simulink library "lib_BuildingThermalLiquid"  (R2026a)
settings: Solver=VariableStepAuto
libraries: ExternalWall_lib x47, WallSelector_lib x36, fl_lib x20, RoomWithRadiatorAndUFP x15
(part 1 of 5)
settings Model: Creator=vikrants  LastModifiedBy=vikrants

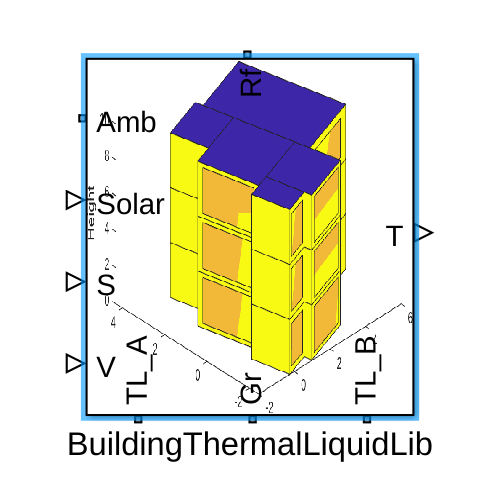
[thumbnail: Simulink's stored preview of the top-level diagram]
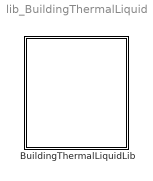
== system lib_BuildingThermalLiquid ==
  BuildingThermalLiquidLib : Subsystem
      settings: PortSchema="{\"entries\":[{\"content\":{\"sides\":[{\"content\":{\"connectorIds\":[\"LConn1\",\"LConn2\",\"LConn3\",\"LConn4\"]},\"type\":\"ConnectorPlacement.EquallySpacedRectSide\",\"uuid\":\"3d4f604e-be28-4e36-924c-1451eaa25fd5\"},{\"content\":{\"connectorIds\":[\"RConn1\"],\"side\":\"RIGHT\"},\"type\":\"ConnectorPlacement.EquallySpacedRectSide\",\"uuid\":\"4c994dcc-0f2c-417a-aef1-7383a3b9052f\"},{\"content\":{\"connectorIds\":[\"LConn5\"],\"side\":\"TOP\"},\"type\":\"ConnectorPlacement.EquallySpacedRectSide\",\"uuid\":\"8e95fada-93f8-47aa-9321-3e2d1640391a\"},{\"content\":{\"connectorIds\":[\"RConn2\",\"RConn3\",\"RConn4\"],\"side\":\"BOTTOM\"},\"type\":\"ConnectorPlacement.EquallySpacedRectSide\",\"uuid\":\"74174f52-ffa4-469a-aac5-7e57a56dc597\"}]},\"type\":\"ConnectorPlacement.EquallySpacedConnector\",\"uuid\":\"f223b6b9-b787-430f-8486-49686756d9cb\"}],\"packageUris\":[\"http://schema.mathworks.com/mf0/Connector/R2020b\"],\"version\":\"1.0\"}"
      mask Display: image('lib_BuildingThermalLiquid.png')

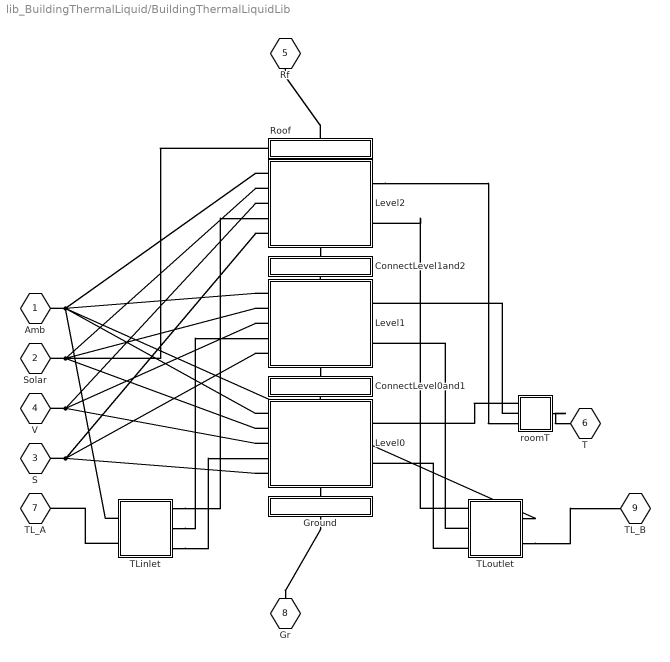
== system lib_BuildingThermalLiquid/BuildingThermalLiquidLib ==
  ConnectLevel0and1 : Subsystem
      settings: PortSchema="{\"entries\":[{\"content\":{\"sides\":[{\"content\":{},\"type\":\"ConnectorPlacement.EquallySpacedRectSide\",\"uuid\":\"f2497a14-4137-415a-aa8b-f8737c2b6cdd\"},{\"content\":{\"side\":\"RIGHT\"},\"type\":\"ConnectorPlacement.EquallySpacedRectSide\",\"uuid\":\"642fe1c4-bc52-48dc-8376-fc1f54abf874\"},{\"content\":{\"connectorIds\":[\"LConn1\"],\"side\":\"TOP\"},\"type\":\"ConnectorPlacement.EquallySpacedRectSide\",\"uuid\":\"0041873e-f83c-4980-a922-5fb2e99c62be\"},{\"content\":{\"connectorIds\":[\"RConn1\"],\"side\":\"BOTTOM\"},\"type\":\"ConnectorPlacement.EquallySpacedRectSide\",\"uuid\":\"519cd5c6-7a50-4e8d-a798-15261cf86acb\"}]},\"type\":\"ConnectorPlacement.EquallySpacedConnector\",\"uuid\":\"f9a0d06d-e057-47b8-97bb-81916403e866\"}],\"packageUris\":[\"http://schema.mathworks.com/mf0/Connector/R2020b\"],\"version\":\"1.0\"}"
  ConnectLevel1and2 : Subsystem
      settings: PortSchema="{\"entries\":[{\"content\":{\"sides\":[{\"content\":{},\"type\":\"ConnectorPlacement.EquallySpacedRectSide\",\"uuid\":\"f2497a14-4137-415a-aa8b-f8737c2b6cdd\"},{\"content\":{\"side\":\"RIGHT\"},\"type\":\"ConnectorPlacement.EquallySpacedRectSide\",\"uuid\":\"642fe1c4-bc52-48dc-8376-fc1f54abf874\"},{\"content\":{\"connectorIds\":[\"LConn1\"],\"side\":\"TOP\"},\"type\":\"ConnectorPlacement.EquallySpacedRectSide\",\"uuid\":\"0041873e-f83c-4980-a922-5fb2e99c62be\"},{\"content\":{\"connectorIds\":[\"RConn1\"],\"side\":\"BOTTOM\"},\"type\":\"ConnectorPlacement.EquallySpacedRectSide\",\"uuid\":\"a780114b-2d0a-4cf5-8292-ebaab293840d\"}]},\"type\":\"ConnectorPlacement.EquallySpacedConnector\",\"uuid\":\"f9a0d06d-e057-47b8-97bb-81916403e866\"}],\"packageUris\":[\"http://schema.mathworks.com/mf0/Connector/R2020b\"],\"version\":\"1.0\"}"
  Ground : Subsystem
      settings: PortSchema="{\"entries\":[{\"content\":{\"sides\":[{\"content\":{},\"type\":\"ConnectorPlacement.EquallySpacedRectSide\",\"uuid\":\"f2497a14-4137-415a-aa8b-f8737c2b6cdd\"},{\"content\":{\"side\":\"RIGHT\"},\"type\":\"ConnectorPlacement.EquallySpacedRectSide\",\"uuid\":\"642fe1c4-bc52-48dc-8376-fc1f54abf874\"},{\"content\":{\"connectorIds\":[\"LConn1\"],\"side\":\"TOP\"},\"type\":\"ConnectorPlacement.EquallySpacedRectSide\",\"uuid\":\"0041873e-f83c-4980-a922-5fb2e99c62be\"},{\"content\":{\"connectorIds\":[\"RConn1\"],\"side\":\"BOTTOM\"},\"type\":\"ConnectorPlacement.EquallySpacedRectSide\",\"uuid\":\"6efa04cd-1264-4f10-80b2-069a220ffbe0\"}]},\"type\":\"ConnectorPlacement.EquallySpacedConnector\",\"uuid\":\"f9a0d06d-e057-47b8-97bb-81916403e866\"}],\"packageUris\":[\"http://schema.mathworks.com/mf0/Connector/R2020b\"],\"version\":\"1.0\"}"
  Level0 : Subsystem
      settings: PortSchema="{\"entries\":[{\"content\":{\"sides\":[{\"content\":{\"connectorIds\":[\"LConn1\",\"LConn2\",\"LConn3\",\"LConn4\",\"LConn5\"]},\"type\":\"ConnectorPlacement.EquallySpacedRectSide\",\"uuid\":\"29492f5e-f304-4ed0-9062-38da432019c8\"},{\"content\":{\"connectorIds\":[\"RConn1\",\"RConn2\"],\"side\":\"RIGHT\"},\"type\":\"ConnectorPlacement.EquallySpacedRectSide\",\"uuid\":\"f46545ef-22ad-458b-9be7-cff6591fe741\"},{\"content\":{\"connectorIds\":[\"LConn6\"],\"side\":\"TOP\"},\"type\":\"ConnectorPlacement.EquallySpacedRectSide\",\"uuid\":\"9b1b30be-62a1-4a86-b987-44a9b36d130d\"},{\"content\":{\"connectorIds\":[\"RConn3\"],\"side\":\"BOTTOM\"},\"type\":\"ConnectorPlacement.EquallySpacedRectSide\",\"uuid\":\"1c461fab-c590-4319-ab41-1586157498f8\"}]},\"type\":\"ConnectorPlacement.EquallySpacedConnector\",\"uuid\":\"6c3f86bb-1201-4f27-98f2-2151c6075667\"}],\"packageUris\":[\"http://schema.mathworks.com/mf0/Connector/R2020b\"],\"version\":\"1.0\"}"
  Level1 : Subsystem
      settings: PortSchema="{\"entries\":[{\"content\":{\"sides\":[{\"content\":{\"connectorIds\":[\"LConn1\",\"LConn2\",\"LConn3\",\"LConn4\",\"LConn5\"]},\"type\":\"ConnectorPlacement.EquallySpacedRectSide\",\"uuid\":\"29492f5e-f304-4ed0-9062-38da432019c8\"},{\"content\":{\"connectorIds\":[\"RConn1\",\"RConn2\"],\"side\":\"RIGHT\"},\"type\":\"ConnectorPlacement.EquallySpacedRectSide\",\"uuid\":\"f46545ef-22ad-458b-9be7-cff6591fe741\"},{\"content\":{\"connectorIds\":[\"LConn6\"],\"side\":\"TOP\"},\"type\":\"ConnectorPlacement.EquallySpacedRectSide\",\"uuid\":\"9b1b30be-62a1-4a86-b987-44a9b36d130d\"},{\"content\":{\"connectorIds\":[\"RConn3\"],\"side\":\"BOTTOM\"},\"type\":\"ConnectorPlacement.EquallySpacedRectSide\",\"uuid\":\"e01c8120-d70d-4a42-a08e-230c171c29be\"}]},\"type\":\"ConnectorPlacement.EquallySpacedConnector\",\"uuid\":\"6c3f86bb-1201-4f27-98f2-2151c6075667\"}],\"packageUris\":[\"http://schema.mathworks.com/mf0/Connector/R2020b\"],\"version\":\"1.0\"}"
  Level2 : Subsystem
      settings: PortSchema="{\"entries\":[{\"content\":{\"sides\":[{\"content\":{\"connectorIds\":[\"LConn1\",\"LConn2\",\"LConn3\",\"LConn4\",\"LConn5\"]},\"type\":\"ConnectorPlacement.EquallySpacedRectSide\",\"uuid\":\"29492f5e-f304-4ed0-9062-38da432019c8\"},{\"content\":{\"connectorIds\":[\"RConn1\",\"RConn2\"],\"side\":\"RIGHT\"},\"type\":\"ConnectorPlacement.EquallySpacedRectSide\",\"uuid\":\"f46545ef-22ad-458b-9be7-cff6591fe741\"},{\"content\":{\"connectorIds\":[\"LConn6\"],\"side\":\"TOP\"},\"type\":\"ConnectorPlacement.EquallySpacedRectSide\",\"uuid\":\"9b1b30be-62a1-4a86-b987-44a9b36d130d\"},{\"content\":{\"connectorIds\":[\"RConn3\"],\"side\":\"BOTTOM\"},\"type\":\"ConnectorPlacement.EquallySpacedRectSide\",\"uuid\":\"fba86260-54d8-4078-9f73-b7a4e9f151fe\"}]},\"type\":\"ConnectorPlacement.EquallySpacedConnector\",\"uuid\":\"6c3f86bb-1201-4f27-98f2-2151c6075667\"}],\"packageUris\":[\"http://schema.mathworks.com/mf0/Connector/R2020b\"],\"version\":\"1.0\"}"
  Roof : Subsystem
      settings: PortSchema="{\"entries\":[{\"content\":{\"sides\":[{\"content\":{\"connectorIds\":[\"LConn1\"]},\"type\":\"ConnectorPlacement.EquallySpacedRectSide\",\"uuid\":\"8a3f7f62-740f-4024-84fd-cea985b0aa8d\"},{\"content\":{\"side\":\"RIGHT\"},\"type\":\"ConnectorPlacement.EquallySpacedRectSide\",\"uuid\":\"b896e2bb-4320-404c-bfaa-2c8ea40bf71f\"},{\"content\":{\"connectorIds\":[\"LConn2\"],\"side\":\"TOP\"},\"type\":\"ConnectorPlacement.EquallySpacedRectSide\",\"uuid\":\"76c3d6f3-9638-4345-911f-6db02cf3c8d9\"},{\"content\":{\"connectorIds\":[\"RConn1\"],\"side\":\"BOTTOM\"},\"type\":\"ConnectorPlacement.EquallySpacedRectSide\",\"uuid\":\"d013c520-b3cf-4758-8021-0d51b5bea7ff\"}]},\"type\":\"ConnectorPlacement.EquallySpacedConnector\",\"uuid\":\"2675eef2-482a-4a5a-91dc-eba58fd9f740\"}],\"packageUris\":[\"http://schema.mathworks.com/mf0/Connector/R2020b\"],\"version\":\"1.0\"}"
  TLinlet : Subsystem
  TLoutlet : Subsystem
  roomT : Subsystem
  Amb : PMIOPort  Side=Left
  Solar : PMIOPort  Port=2  Side=Left
  S : PMIOPort  Port=3  Side=Left
  V : PMIOPort  Port=4  Side=Left
  Rf : PMIOPort  Port=5  Side=Left
  T : PMIOPort  Port=6  Side=Right
  TL_A : PMIOPort  Port=7  Side=Right
  Gr : PMIOPort  Port=8  Side=Right
  TL_B : PMIOPort  Port=9  Side=Right
  connections:
  TLinlet/RConn1 -- Level2/LConn4
  TLoutlet/LConn1 -- Level2/RConn2
  TLinlet/RConn2 -- Level1/LConn4
  TLoutlet/LConn2 -- Level1/RConn2
  TLinlet/RConn3 -- Level0/LConn4
  TLoutlet/LConn3 -- Level0/RConn2
  Level0/RConn3 -- Ground/LConn1
  Level1/RConn3 -- ConnectLevel0and1/LConn1
  Level0/LConn6 -- ConnectLevel0and1/RConn1
  Level2/RConn3 -- ConnectLevel1and2/LConn1
  Level1/LConn6 -- ConnectLevel1and2/RConn1
  Level2/LConn6 -- Roof/RConn1
  Roof/LConn2 -- Rf/RConn1
  Ground/RConn1 -- Gr/RConn1
  Roof/LConn1 -- Solar/RConn1 -- Level2/LConn2 -- Level1/LConn2 -- Level0/LConn2
  Level0/LConn1 -- Amb/RConn1 -- TLoutlet/RConn1 -- TLinlet/LConn1 -- Level2/LConn1 -- Level1/LConn1
  Level0/LConn3 -- V/RConn1 -- Level2/LConn3 -- Level1/LConn3
  Level0/LConn5 -- S/RConn1 -- Level2/LConn5 -- Level1/LConn5
  TLinlet/LConn2 -- TL_A/RConn1
  TLoutlet/RConn2 -- TL_B/RConn1
  roomT/LConn2 -- Level1/RConn1
  roomT/RConn1 -- T/RConn1
  roomT/LConn1 -- Level0/RConn1
  Level2/RConn1 -- roomT/LConn3

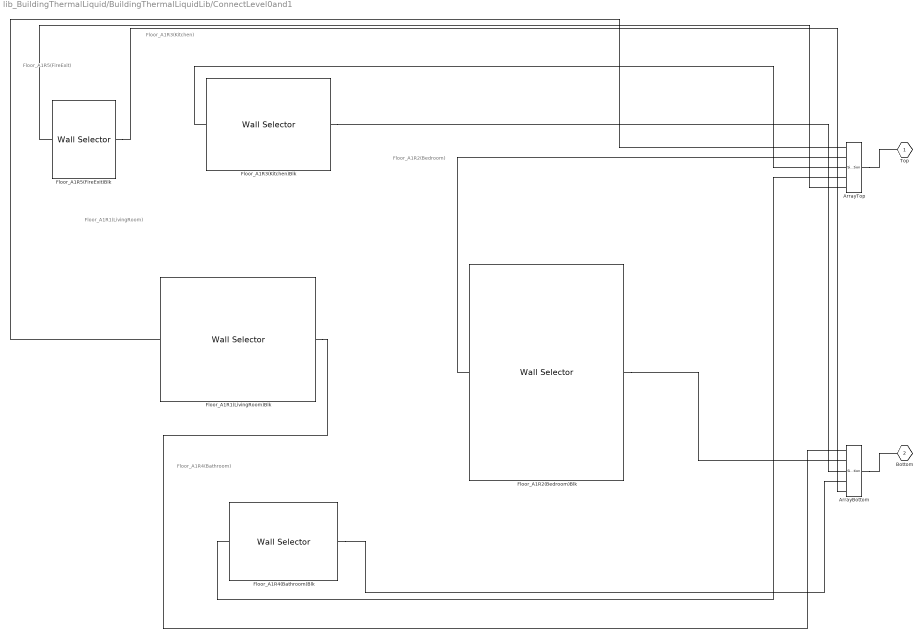
== system lib_BuildingThermalLiquid/BuildingThermalLiquidLib/ConnectLevel0and1 ==
  note: Floor_A1R1(LivingRoom)
  note: Floor_A1R2(Bedroom)
  note: Floor_A1R3(Kitchen)
  note: Floor_A1R4(Bathroom)
  note: Floor_A1R5(FireExit)
  ArrayBottom : SimscapeArrayConnection  Domain=foundation.thermal.thermal  ConcatenateDimension=1  NumScalarElements=5
  ArrayTop : SimscapeArrayConnection  Domain=foundation.thermal.thermal  ConcatenateDimension=1  NumScalarElements=5
  Floor_A1R1(LivingRoom)Blk : WallSelector_lib/Wall Selector  optWall=wallModelOption.wallOnly  wallLength=2.4384 % Parameterized on : 11-Dec-2025 09:25:46 m  wallHeight=3.048 % Parameterized on : 11-Dec-2025 09:25:46 m  wallThickness=0.03 % Parameterized on : 11-Dec-2025 09:25:46 m  wallMaterialDen=1400 % Parameterized on : 11-Dec-2025 09:25:49 kg/m^3  wallMaterialCp=1000 % Parameterized on : 11-Dec-2025 09:25:49 J/(K*kg)  wallAbsorptivity=0.5  wallThermalK=0.7 % Parameterized on : 11-Dec-2025 09:25:49 W/(K*m)  winLength=1 m  winHeight=0.5 m  winThickness=0.007 m  winMaterialDen=2500 kg/m^3  winMaterialCp=787 J/(K*kg)  winAbsorptivity=0.35  winThermalK=1 W/(K*m)  winTransmissivity=0.45  ventLength=0.1 m  ventHeight=0.1 m  extToWallHTC=30 % Parameterized on : 11-Dec-2025 09:25:49 W/(K*m^2)  intToRoomHTC=30 % Parameterized on : 11-Dec-2025 09:25:49 W/(K*m^2)  iniT=300 % Parameterized on : 11-Dec-2025 09:25:49 K
  Floor_A1R2(Bedroom)Blk : WallSelector_lib/Wall Selector  optWall=wallModelOption.wallOnly  wallLength=4.2672 % Parameterized on : 11-Dec-2025 09:25:46 m  wallHeight=3.048 % Parameterized on : 11-Dec-2025 09:25:46 m  wallThickness=0.03 % Parameterized on : 11-Dec-2025 09:25:46 m  wallMaterialDen=1400 % Parameterized on : 11-Dec-2025 09:25:49 kg/m^3  wallMaterialCp=1000 % Parameterized on : 11-Dec-2025 09:25:49 J/(K*kg)  wallAbsorptivity=0.5  wallThermalK=0.7 % Parameterized on : 11-Dec-2025 09:25:49 W/(K*m)  winLength=1 m  winHeight=0.5 m  winThickness=0.007 m  winMaterialDen=2500 kg/m^3  winMaterialCp=787 J/(K*kg)  winAbsorptivity=0.35  winThermalK=1 W/(K*m)  winTransmissivity=0.45  ventLength=0.1 m  ventHeight=0.1 m  extToWallHTC=30 % Parameterized on : 11-Dec-2025 09:25:49 W/(K*m^2)  intToRoomHTC=30 % Parameterized on : 11-Dec-2025 09:25:49 W/(K*m^2)  iniT=300 % Parameterized on : 11-Dec-2025 09:25:49 K
  Floor_A1R3(Kitchen)Blk : WallSelector_lib/Wall Selector  optWall=wallModelOption.wallOnly  wallLength=1.8288 % Parameterized on : 11-Dec-2025 09:25:46 m  wallHeight=2.4384 % Parameterized on : 11-Dec-2025 09:25:46 m  wallThickness=0.03 % Parameterized on : 11-Dec-2025 09:25:46 m  wallMaterialDen=1400 % Parameterized on : 11-Dec-2025 09:25:49 kg/m^3  wallMaterialCp=1000 % Parameterized on : 11-Dec-2025 09:25:49 J/(K*kg)  wallAbsorptivity=0.5  wallThermalK=0.7 % Parameterized on : 11-Dec-2025 09:25:49 W/(K*m)  winLength=1 m  winHeight=0.5 m  winThickness=0.007 m  winMaterialDen=2500 kg/m^3  winMaterialCp=787 J/(K*kg)  winAbsorptivity=0.35  winThermalK=1 W/(K*m)  winTransmissivity=0.45  ventLength=0.1 m  ventHeight=0.1 m  extToWallHTC=30 % Parameterized on : 11-Dec-2025 09:25:49 W/(K*m^2)  intToRoomHTC=30 % Parameterized on : 11-Dec-2025 09:25:49 W/(K*m^2)  iniT=300 % Parameterized on : 11-Dec-2025 09:25:49 K
  Floor_A1R4(Bathroom)Blk : WallSelector_lib/Wall Selector  optWall=wallModelOption.wallOnly  wallLength=1.524 % Parameterized on : 11-Dec-2025 09:25:46 m  wallHeight=2.1336 % Parameterized on : 11-Dec-2025 09:25:47 m  wallThickness=0.03 % Parameterized on : 11-Dec-2025 09:25:47 m  wallMaterialDen=1400 % Parameterized on : 11-Dec-2025 09:25:49 kg/m^3  wallMaterialCp=1000 % Parameterized on : 11-Dec-2025 09:25:49 J/(K*kg)  wallAbsorptivity=0.5  wallThermalK=0.7 % Parameterized on : 11-Dec-2025 09:25:49 W/(K*m)  winLength=1 m  winHeight=0.5 m  winThickness=0.007 m  winMaterialDen=2500 kg/m^3  winMaterialCp=787 J/(K*kg)  winAbsorptivity=0.35  winThermalK=1 W/(K*m)  winTransmissivity=0.45  ventLength=0.1 m  ventHeight=0.1 m  extToWallHTC=30 % Parameterized on : 11-Dec-2025 09:25:49 W/(K*m^2)  intToRoomHTC=30 % Parameterized on : 11-Dec-2025 09:25:49 W/(K*m^2)  iniT=300 % Parameterized on : 11-Dec-2025 09:25:49 K
  Floor_A1R5(FireExit)Blk : WallSelector_lib/Wall Selector  optWall=wallModelOption.wallOnly  wallLength=1.524 % Parameterized on : 11-Dec-2025 09:25:47 m  wallHeight=1.2192 % Parameterized on : 11-Dec-2025 09:25:47 m  wallThickness=0.03 % Parameterized on : 11-Dec-2025 09:25:47 m  wallMaterialDen=1400 % Parameterized on : 11-Dec-2025 09:25:49 kg/m^3  wallMaterialCp=1000 % Parameterized on : 11-Dec-2025 09:25:49 J/(K*kg)  wallAbsorptivity=0.5  wallThermalK=0.7 % Parameterized on : 11-Dec-2025 09:25:49 W/(K*m)  winLength=1 m  winHeight=0.5 m  winThickness=0.007 m  winMaterialDen=2500 kg/m^3  winMaterialCp=787 J/(K*kg)  winAbsorptivity=0.35  winThermalK=1 W/(K*m)  winTransmissivity=0.45  ventLength=0.1 m  ventHeight=0.1 m  extToWallHTC=30 % Parameterized on : 11-Dec-2025 09:25:49 W/(K*m^2)  intToRoomHTC=30 % Parameterized on : 11-Dec-2025 09:25:49 W/(K*m^2)  iniT=300 % Parameterized on : 11-Dec-2025 09:25:49 K
  Top : PMIOPort  Side=Left
  Bottom : PMIOPort  Port=2  Side=Right
  connections:
  ArrayTop/RConn1 -- Top/RConn1
  Floor_A1R1(LivingRoom)Blk/LConn1 -- ArrayTop/LConn1
  Floor_A1R2(Bedroom)Blk/LConn1 -- ArrayTop/LConn2
  Floor_A1R3(Kitchen)Blk/LConn1 -- ArrayTop/LConn3
  Floor_A1R4(Bathroom)Blk/LConn1 -- ArrayTop/LConn4
  Floor_A1R5(FireExit)Blk/LConn1 -- ArrayTop/LConn5
  ArrayBottom/RConn1 -- Bottom/RConn1
  Floor_A1R1(LivingRoom)Blk/RConn1 -- ArrayBottom/LConn1
  Floor_A1R2(Bedroom)Blk/RConn1 -- ArrayBottom/LConn2
  Floor_A1R3(Kitchen)Blk/RConn1 -- ArrayBottom/LConn3
  Floor_A1R4(Bathroom)Blk/RConn1 -- ArrayBottom/LConn4
  Floor_A1R5(FireExit)Blk/RConn1 -- ArrayBottom/LConn5

== system lib_BuildingThermalLiquid/BuildingThermalLiquidLib/ConnectLevel1and2 ==
  note: Floor_A2R1(LivingRoom)
  note: Floor_A2R2(Bedroom)
  note: Floor_A2R3(Kitchen)
  note: Floor_A2R4(Bathroom)
  note: Floor_A2R5(FireExit)
  ArrayBottom : SimscapeArrayConnection  Domain=foundation.thermal.thermal  ConcatenateDimension=1  NumScalarElements=5
  ArrayTop : SimscapeArrayConnection  Domain=foundation.thermal.thermal  ConcatenateDimension=1  NumScalarElements=5
  Floor_A2R1(LivingRoom)Blk : WallSelector_lib/Wall Selector  optWall=wallModelOption.wallOnly  wallLength=2.4384 % Parameterized on : 11-Dec-2025 09:25:47 m  wallHeight=3.048 % Parameterized on : 11-Dec-2025 09:25:47 m  wallThickness=0.03 % Parameterized on : 11-Dec-2025 09:25:47 m  wallMaterialDen=1400 % Parameterized on : 11-Dec-2025 09:25:49 kg/m^3  wallMaterialCp=1000 % Parameterized on : 11-Dec-2025 09:25:49 J/(K*kg)  wallAbsorptivity=0.5  wallThermalK=0.7 % Parameterized on : 11-Dec-2025 09:25:49 W/(K*m)  winLength=1 m  winHeight=0.5 m  winThickness=0.007 m  winMaterialDen=2500 kg/m^3  winMaterialCp=787 J/(K*kg)  winAbsorptivity=0.35  winThermalK=1 W/(K*m)  winTransmissivity=0.45  ventLength=0.1 m  ventHeight=0.1 m  extToWallHTC=30 % Parameterized on : 11-Dec-2025 09:25:49 W/(K*m^2)  intToRoomHTC=30 % Parameterized on : 11-Dec-2025 09:25:49 W/(K*m^2)  iniT=300 % Parameterized on : 11-Dec-2025 09:25:49 K
  Floor_A2R2(Bedroom)Blk : WallSelector_lib/Wall Selector  optWall=wallModelOption.wallOnly  wallLength=4.2672 % Parameterized on : 11-Dec-2025 09:25:47 m  wallHeight=3.048 % Parameterized on : 11-Dec-2025 09:25:47 m  wallThickness=0.03 % Parameterized on : 11-Dec-2025 09:25:47 m  wallMaterialDen=1400 % Parameterized on : 11-Dec-2025 09:25:49 kg/m^3  wallMaterialCp=1000 % Parameterized on : 11-Dec-2025 09:25:49 J/(K*kg)  wallAbsorptivity=0.5  wallThermalK=0.7 % Parameterized on : 11-Dec-2025 09:25:49 W/(K*m)  winLength=1 m  winHeight=0.5 m  winThickness=0.007 m  winMaterialDen=2500 kg/m^3  winMaterialCp=787 J/(K*kg)  winAbsorptivity=0.35  winThermalK=1 W/(K*m)  winTransmissivity=0.45  ventLength=0.1 m  ventHeight=0.1 m  extToWallHTC=30 % Parameterized on : 11-Dec-2025 09:25:49 W/(K*m^2)  intToRoomHTC=30 % Parameterized on : 11-Dec-2025 09:25:49 W/(K*m^2)  iniT=300 % Parameterized on : 11-Dec-2025 09:25:49 K
  Floor_A2R3(Kitchen)Blk : WallSelector_lib/Wall Selector  optWall=wallModelOption.wallOnly  wallLength=1.8288 % Parameterized on : 11-Dec-2025 09:25:47 m  wallHeight=2.4384 % Parameterized on : 11-Dec-2025 09:25:47 m  wallThickness=0.03 % Parameterized on : 11-Dec-2025 09:25:47 m  wallMaterialDen=1400 % Parameterized on : 11-Dec-2025 09:25:49 kg/m^3  wallMaterialCp=1000 % Parameterized on : 11-Dec-2025 09:25:49 J/(K*kg)  wallAbsorptivity=0.5  wallThermalK=0.7 % Parameterized on : 11-Dec-2025 09:25:49 W/(K*m)  winLength=1 m  winHeight=0.5 m  winThickness=0.007 m  winMaterialDen=2500 kg/m^3  winMaterialCp=787 J/(K*kg)  winAbsorptivity=0.35  winThermalK=1 W/(K*m)  winTransmissivity=0.45  ventLength=0.1 m  ventHeight=0.1 m  extToWallHTC=30 % Parameterized on : 11-Dec-2025 09:25:49 W/(K*m^2)  intToRoomHTC=30 % Parameterized on : 11-Dec-2025 09:25:49 W/(K*m^2)  iniT=300 % Parameterized on : 11-Dec-2025 09:25:49 K
  Floor_A2R4(Bathroom)Blk : WallSelector_lib/Wall Selector  optWall=wallModelOption.wallOnly  wallLength=1.524 % Parameterized on : 11-Dec-2025 09:25:47 m  wallHeight=2.1336 % Parameterized on : 11-Dec-2025 09:25:47 m  wallThickness=0.03 % Parameterized on : 11-Dec-2025 09:25:47 m  wallMaterialDen=1400 % Parameterized on : 11-Dec-2025 09:25:49 kg/m^3  wallMaterialCp=1000 % Parameterized on : 11-Dec-2025 09:25:49 J/(K*kg)  wallAbsorptivity=0.5  wallThermalK=0.7 % Parameterized on : 11-Dec-2025 09:25:49 W/(K*m)  winLength=1 m  winHeight=0.5 m  winThickness=0.007 m  winMaterialDen=2500 kg/m^3  winMaterialCp=787 J/(K*kg)  winAbsorptivity=0.35  winThermalK=1 W/(K*m)  winTransmissivity=0.45  ventLength=0.1 m  ventHeight=0.1 m  extToWallHTC=30 % Parameterized on : 11-Dec-2025 09:25:49 W/(K*m^2)  intToRoomHTC=30 % Parameterized on : 11-Dec-2025 09:25:49 W/(K*m^2)  iniT=300 % Parameterized on : 11-Dec-2025 09:25:49 K
  Floor_A2R5(FireExit)Blk : WallSelector_lib/Wall Selector  optWall=wallModelOption.wallOnly  wallLength=1.524 % Parameterized on : 11-Dec-2025 09:25:47 m  wallHeight=1.2192 % Parameterized on : 11-Dec-2025 09:25:47 m  wallThickness=0.03 % Parameterized on : 11-Dec-2025 09:25:47 m  wallMaterialDen=1400 % Parameterized on : 11-Dec-2025 09:25:49 kg/m^3  wallMaterialCp=1000 % Parameterized on : 11-Dec-2025 09:25:49 J/(K*kg)  wallAbsorptivity=0.5  wallThermalK=0.7 % Parameterized on : 11-Dec-2025 09:25:49 W/(K*m)  winLength=1 m  winHeight=0.5 m  winThickness=0.007 m  winMaterialDen=2500 kg/m^3  winMaterialCp=787 J/(K*kg)  winAbsorptivity=0.35  winThermalK=1 W/(K*m)  winTransmissivity=0.45  ventLength=0.1 m  ventHeight=0.1 m  extToWallHTC=30 % Parameterized on : 11-Dec-2025 09:25:49 W/(K*m^2)  intToRoomHTC=30 % Parameterized on : 11-Dec-2025 09:25:49 W/(K*m^2)  iniT=300 % Parameterized on : 11-Dec-2025 09:25:49 K
  Top : PMIOPort  Side=Left
  Bottom : PMIOPort  Port=2  Side=Right
  connections:
  ArrayTop/RConn1 -- Top/RConn1
  Floor_A2R1(LivingRoom)Blk/LConn1 -- ArrayTop/LConn1
  Floor_A2R2(Bedroom)Blk/LConn1 -- ArrayTop/LConn2
  Floor_A2R3(Kitchen)Blk/LConn1 -- ArrayTop/LConn3
  Floor_A2R4(Bathroom)Blk/LConn1 -- ArrayTop/LConn4
  Floor_A2R5(FireExit)Blk/LConn1 -- ArrayTop/LConn5
  ArrayBottom/RConn1 -- Bottom/RConn1
  Floor_A2R1(LivingRoom)Blk/RConn1 -- ArrayBottom/LConn1
  Floor_A2R2(Bedroom)Blk/RConn1 -- ArrayBottom/LConn2
  Floor_A2R3(Kitchen)Blk/RConn1 -- ArrayBottom/LConn3
  Floor_A2R4(Bathroom)Blk/RConn1 -- ArrayBottom/LConn4
  Floor_A2R5(FireExit)Blk/RConn1 -- ArrayBottom/LConn5

== system lib_BuildingThermalLiquid/BuildingThermalLiquidLib/Ground ==
  note: Ground_A1R1(LivingRoom)
  note: Ground_A1R2(Bedroom)
  note: Ground_A1R3(Kitchen)
  note: Ground_A1R4(Bathroom)
  note: Ground_A1R5(FireExit)
  ArrayBottom : SimscapeArrayConnection  Domain=foundation.thermal.thermal  ConcatenateDimension=1  NumScalarElements=5
  ArrayTop : SimscapeArrayConnection  Domain=foundation.thermal.thermal  ConcatenateDimension=1  NumScalarElements=5
  Ground_A1R1(LivingRoom)Blk : WallSelector_lib/Wall Selector  optWall=wallModelOption.wallOnly  wallLength=2.4384 % Parameterized on : 11-Dec-2025 09:25:47 m  wallHeight=3.048 % Parameterized on : 11-Dec-2025 09:25:47 m  wallThickness=0.03 % Parameterized on : 11-Dec-2025 09:25:47 m  wallMaterialDen=1400 % Parameterized on : 11-Dec-2025 09:25:49 kg/m^3  wallMaterialCp=1000 % Parameterized on : 11-Dec-2025 09:25:49 J/(K*kg)  wallAbsorptivity=0.5  wallThermalK=0.7 % Parameterized on : 11-Dec-2025 09:25:49 W/(K*m)  winLength=1 m  winHeight=0.5 m  winThickness=0.007 m  winMaterialDen=2500 kg/m^3  winMaterialCp=787 J/(K*kg)  winAbsorptivity=0.35  winThermalK=1 W/(K*m)  winTransmissivity=0.45  ventLength=0.1 m  ventHeight=0.1 m  extToWallHTC=30 % Parameterized on : 11-Dec-2025 09:25:49 W/(K*m^2)  intToRoomHTC=30 % Parameterized on : 11-Dec-2025 09:25:49 W/(K*m^2)  iniT=300 % Parameterized on : 11-Dec-2025 09:25:49 K
  Ground_A1R2(Bedroom)Blk : WallSelector_lib/Wall Selector  optWall=wallModelOption.wallOnly  wallLength=4.2672 % Parameterized on : 11-Dec-2025 09:25:47 m  wallHeight=3.048 % Parameterized on : 11-Dec-2025 09:25:47 m  wallThickness=0.03 % Parameterized on : 11-Dec-2025 09:25:47 m  wallMaterialDen=1400 % Parameterized on : 11-Dec-2025 09:25:49 kg/m^3  wallMaterialCp=1000 % Parameterized on : 11-Dec-2025 09:25:49 J/(K*kg)  wallAbsorptivity=0.5  wallThermalK=0.7 % Parameterized on : 11-Dec-2025 09:25:49 W/(K*m)  winLength=1 m  winHeight=0.5 m  winThickness=0.007 m  winMaterialDen=2500 kg/m^3  winMaterialCp=787 J/(K*kg)  winAbsorptivity=0.35  winThermalK=1 W/(K*m)  winTransmissivity=0.45  ventLength=0.1 m  ventHeight=0.1 m  extToWallHTC=30 % Parameterized on : 11-Dec-2025 09:25:49 W/(K*m^2)  intToRoomHTC=30 % Parameterized on : 11-Dec-2025 09:25:49 W/(K*m^2)  iniT=300 % Parameterized on : 11-Dec-2025 09:25:49 K
  Ground_A1R3(Kitchen)Blk : WallSelector_lib/Wall Selector  optWall=wallModelOption.wallOnly  wallLength=1.8288 % Parameterized on : 11-Dec-2025 09:25:47 m  wallHeight=2.4384 % Parameterized on : 11-Dec-2025 09:25:47 m  wallThickness=0.03 % Parameterized on : 11-Dec-2025 09:25:47 m  wallMaterialDen=1400 % Parameterized on : 11-Dec-2025 09:25:49 kg/m^3  wallMaterialCp=1000 % Parameterized on : 11-Dec-2025 09:25:49 J/(K*kg)  wallAbsorptivity=0.5  wallThermalK=0.7 % Parameterized on : 11-Dec-2025 09:25:49 W/(K*m)  winLength=1 m  winHeight=0.5 m  winThickness=0.007 m  winMaterialDen=2500 kg/m^3  winMaterialCp=787 J/(K*kg)  winAbsorptivity=0.35  winThermalK=1 W/(K*m)  winTransmissivity=0.45  ventLength=0.1 m  ventHeight=0.1 m  extToWallHTC=30 % Parameterized on : 11-Dec-2025 09:25:49 W/(K*m^2)  intToRoomHTC=30 % Parameterized on : 11-Dec-2025 09:25:49 W/(K*m^2)  iniT=300 % Parameterized on : 11-Dec-2025 09:25:49 K
  Ground_A1R4(Bathroom)Blk : WallSelector_lib/Wall Selector  optWall=wallModelOption.wallOnly  wallLength=1.524 % Parameterized on : 11-Dec-2025 09:25:47 m  wallHeight=2.1336 % Parameterized on : 11-Dec-2025 09:25:47 m  wallThickness=0.03 % Parameterized on : 11-Dec-2025 09:25:47 m  wallMaterialDen=1400 % Parameterized on : 11-Dec-2025 09:25:49 kg/m^3  wallMaterialCp=1000 % Parameterized on : 11-Dec-2025 09:25:49 J/(K*kg)  wallAbsorptivity=0.5  wallThermalK=0.7 % Parameterized on : 11-Dec-2025 09:25:49 W/(K*m)  winLength=1 m  winHeight=0.5 m  winThickness=0.007 m  winMaterialDen=2500 kg/m^3  winMaterialCp=787 J/(K*kg)  winAbsorptivity=0.35  winThermalK=1 W/(K*m)  winTransmissivity=0.45  ventLength=0.1 m  ventHeight=0.1 m  extToWallHTC=30 % Parameterized on : 11-Dec-2025 09:25:49 W/(K*m^2)  intToRoomHTC=30 % Parameterized on : 11-Dec-2025 09:25:49 W/(K*m^2)  iniT=300 % Parameterized on : 11-Dec-2025 09:25:49 K
  Ground_A1R5(FireExit)Blk : WallSelector_lib/Wall Selector  optWall=wallModelOption.wallOnly  wallLength=1.524 % Parameterized on : 11-Dec-2025 09:25:47 m  wallHeight=1.2192 % Parameterized on : 11-Dec-2025 09:25:47 m  wallThickness=0.03 % Parameterized on : 11-Dec-2025 09:25:47 m  wallMaterialDen=1400 % Parameterized on : 11-Dec-2025 09:25:49 kg/m^3  wallMaterialCp=1000 % Parameterized on : 11-Dec-2025 09:25:49 J/(K*kg)  wallAbsorptivity=0.5  wallThermalK=0.7 % Parameterized on : 11-Dec-2025 09:25:49 W/(K*m)  winLength=1 m  winHeight=0.5 m  winThickness=0.007 m  winMaterialDen=2500 kg/m^3  winMaterialCp=787 J/(K*kg)  winAbsorptivity=0.35  winThermalK=1 W/(K*m)  winTransmissivity=0.45  ventLength=0.1 m  ventHeight=0.1 m  extToWallHTC=30 % Parameterized on : 11-Dec-2025 09:25:49 W/(K*m^2)  intToRoomHTC=30 % Parameterized on : 11-Dec-2025 09:25:49 W/(K*m^2)  iniT=300 % Parameterized on : 11-Dec-2025 09:25:49 K
  Top : PMIOPort  Side=Left
  Bottom : PMIOPort  Port=2  Side=Right
  connections:
  ArrayTop/RConn1 -- Top/RConn1
  Ground_A1R1(LivingRoom)Blk/LConn1 -- ArrayTop/LConn1
  Ground_A1R2(Bedroom)Blk/LConn1 -- ArrayTop/LConn2
  Ground_A1R3(Kitchen)Blk/LConn1 -- ArrayTop/LConn3
  Ground_A1R4(Bathroom)Blk/LConn1 -- ArrayTop/LConn4
  Ground_A1R5(FireExit)Blk/LConn1 -- ArrayTop/LConn5
  ArrayBottom/RConn1 -- Bottom/RConn1
  Ground_A1R1(LivingRoom)Blk/RConn1 -- ArrayBottom/LConn1
  Ground_A1R2(Bedroom)Blk/RConn1 -- ArrayBottom/LConn2
  Ground_A1R3(Kitchen)Blk/RConn1 -- ArrayBottom/LConn3
  Ground_A1R4(Bathroom)Blk/RConn1 -- ArrayBottom/LConn4
  Ground_A1R5(FireExit)Blk/RConn1 -- ArrayBottom/LConn5
